simulink model "LinearActiveSuspension"  (R2018b)
settings: Solver=VariableStepAuto  StartTime=0.0  StopTime=tmax  FixedStep=0.001  RelTol=1e-3
values from neighbouring files (symbols this model uses):
  A = [  0       1         0          -1 ... (first row only)    [load_params.m]
  B = [    0        0 ... (first row only)    [load_params.m]
  C = [   1      0     0     0 ... (first row only)    [load_params.m]
  D = [ 0   0 ... (first row only)    [load_params.m]
settings Model: Creator=alexj  LastModifiedBy=alexj

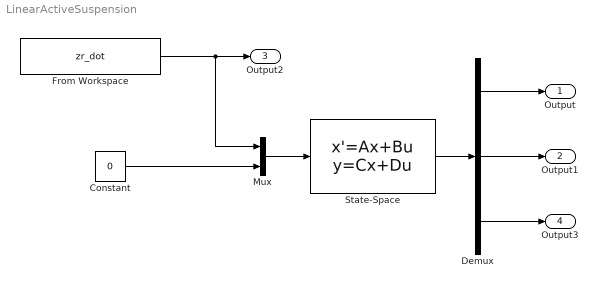
== system LinearActiveSuspension ==
  Constant : Constant  Value=0
  Demux : Demux  Outputs=3
  From Workspace : FromWorkspace  VariableName=zr_dot  SampleTime=0.02  OutputAfterFinalValue=Setting to zero
  Mux : Mux  Inputs=2
  State-Space : StateSpace  A=A  B=B  C=C  D=D  InitialCondition=[0.001 -0.03 -0.016 -0.08]  ContinuousStateAttributes="\"\""
  Output : Outport  SignalName=suspension_travel
  Output1 : Outport  Port=2  SignalName=body_acc
  Output2 : Outport  Port=3  SignalName=zr_dot
  Output3 : Outport  Port=4  SignalName=tire_displacement
  wires:
  Mux/1 -> State-Space/1
  State-Space/1 -> Demux/1
  Demux/1 -> Output/1
  Demux/2 -> Output1/1
  Constant/1 -> Mux/2
  Demux/3 -> Output3/1
  From Workspace/1 -> Mux/1, Output2/1
